simulink model "spiral_karno"  (R2017b)
settings: Solver=VariableStepAuto  StartTime=0.0  StopTime=3  RelTol=1e-4
undefined symbols (not defined in the file or in its folder): magnitude
libraries: simulink x2
settings Model: Creator=user  LastModifiedBy=user

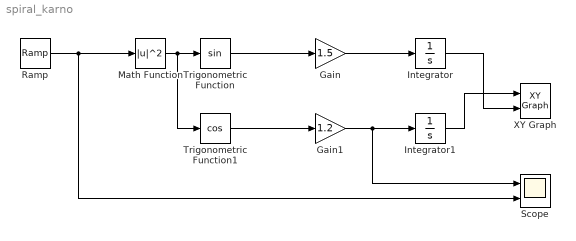
== system spiral_karno ==
  Gain : Gain  Gain=1.5
  Gain1 : Gain  Gain=1.2
  Integrator : Integrator
  Integrator1 : Integrator
  Math Function : Math  Operator=magnitude^2  SaturateOnIntegerOverflow=on
  Ramp : simulink/Sources/Ramp  slope=10  start=0  X0=-20
  Scope : Scope  NumInputPorts=2
  Trigonometric Function : Trigonometry
  Trigonometric Function1 : Trigonometry  Operator=cos
  XY Graph : simulink/Sinks/XY Graph  xmin=-0.5  xmax=0.5  ymin=-0.5  ymax=0.5  st=0.0001
  wires:
  Gain/1 -> Integrator/1
  Trigonometric Function1/1 -> Gain1/1
  Trigonometric Function/1 -> Gain/1
  Gain1/1 -> Scope/1, Integrator1/1
  Ramp/1 -> Math Function/1, Scope/2
  Math Function/1 -> Trigonometric Function1/1, Trigonometric Function/1
  Integrator/1 -> XY Graph/2
  Integrator1/1 -> XY Graph/1
